simulink model "PIDcontinuo"  (R2021a)
settings: Solver=VariableStepAuto  StartTime=0.0  StopTime=10*ts  RelTol=1e-3
values from neighbouring files (symbols this model uses):
  g = 9.81    [Parcial2PIDContinuo.m]
  L = 0.25    [Parcial2PIDContinuo.m]
  m = 0.03    [Parcial2PIDContinuo.m]
  M = 0.510    (= 0.51)    [Parcial2PIDContinuo.m]
  ts = 5    [Parcial2PIDContinuo.m]
libraries: pid_lib x2, spsStairGeneratorLib x1
settings Model: Creator=manue  LastModifiedBy=manue

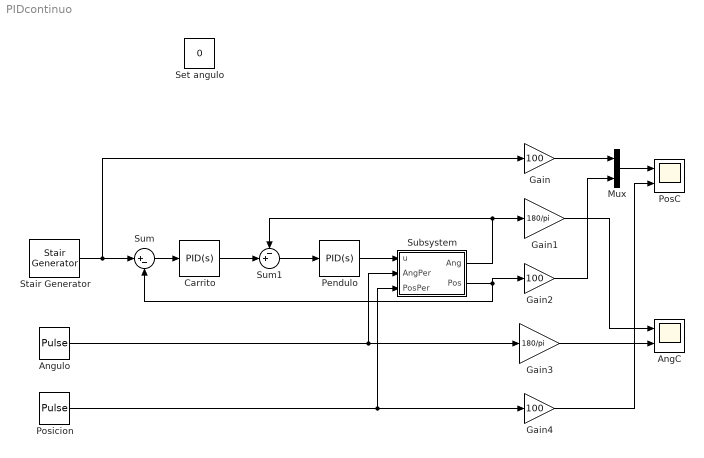
== system PIDcontinuo ==
  AngC : Scope  NumInputPorts=2
  Angulo : DiscretePulseGenerator  PulseType=Time based  Amplitude=10*pi/180  Period=60  PulseWidth=0.1  PhaseDelay=40
  Carrito : pid_lib/PID Controller  Controller=PID  Form=Ideal  TimeDomain=Continuous-time  UseExternalTs=off  SampleTime=-1  IntegratorMethod=Forward Euler  FilterMethod=Forward Euler  ControllerParametersSource=internal  P=0.0857737044561583  I=0.0832220773397635  D=1.96746042698113  UseFilter=on  N=7.47498988089675  TunerSelectOption=Transfer Function Based (PID Tuner App)  InitialConditionSource=internal  InitialConditionForIntegrator=0  InitialConditionForFilter=0  DifferentiatorICPrevScaledInput=0  ExternalReset=none  TrackingMode=off  Kt=1  LimitOutput=off  SatLimitsSource=internal  UpperSaturationLimit=inf  LowerSaturationLimit=-inf  LinearizeAsGain=on  AntiWindupMode=none  Kb=1  POutMin=[]  POutMax=[]  IOutMin=[]  IOutMax=[]  DOutMin=[]  DOutMax=[]  NOutMin=[]  NOutMax=[]  SumOutMin=[]  SumOutMax=[]  SaturationOutMin=[]  SaturationOutMax=[]  PParamMin=[]  PParamMax=[]  IParamMin=[]  IParamMax=[]  DParamMin=[]  DParamMax=[]  NParamMin=[]  NParamMax=[]  KbParamMin=[]  KbParamMax=[]  KtParamMin=[]  KtParamMax=[]  KbOutMin=[]  KbOutMax=[]  KtOutMin=[]  KtOutMax=[]  IntegratorOutMin=[]  IntegratorOutMax=[]  FilterOutMin=[]  FilterOutMax=[]  SumI1OutMin=[]  SumI1OutMax=[]  SumI2OutMin=[]  SumI2OutMax=[]  SumI3OutMin=[]  SumI3OutMax=[]  SumI4OutMin=[]  SumI4OutMax=[]  SumDOutMin=[]  SumDOutMax=[]  DifferentiatorOutMin=[]  DifferentiatorOutMax=[]  FilterDiffOutCoefMin=[]  FilterDiffOutCoefMax=[]  ReciprocalOutMin=[]  ReciprocalOutMax=[]  SumDenOutMin=[]  SumDenOutMax=[]  SumNumOutMin=[]  SumNumOutMax=[]  DivideOutMin=[]  DivideOutMax=[]  UdiffTsProdOutMin=[]  UdiffTsProdOutMax=[]  NTsProdOutMin=[]  NTsProdOutMax=[]  UintegralTsProdOutMin=[]  UintegralTsProdOutMax=[]  UngainTsProdOutMin=[]  UngainTsProdOutMax=[]  IntegratorContinuousStateAttributes=''  IntegratorStateMustResolveToSignalObject=off  IntegratorRTWStateStorageClass=Auto  FilterContinuousStateAttributes=''  FilterStateMustResolveToSignalObject=off  FilterRTWStateStorageClass=Auto  ParallelPVariant=Passthrough  IdealPVariant=InternalParameters  IVariant=InternalParameters  DVariant=InternalParameters  IntegratorVariant=Continuous  SatVariant=Disabled  AWVariant=Passthrough  PCopyVariant=Disabled  TRVariant=Disabled  FdbkBlocksVariant=Forward  IdealPFdbkVariant=Disabled  SatFdbkVariant=Disabled  DerivativeFilterVariant=ContFilter  NVariant=InternalParameters  NCopyVariant=Disabled  FilterICVariant=InternalICsFilter  IntegratorICVariant=InternalICs  ExternalResetVariant=Disabled  TRSumVariant=Passthrough  SumFdbkVariant=Disabled  SumVariant=Sum_PID  TsampFilterVariant=InternalTs  TsampNgainVariant=Passthrough  TsampIntegralVariant=Passthrough  ExternalSaturationOutDataTypeStr=Inherit: Same as second input
  Gain : Gain  Gain=100
  Gain1 : Gain  Gain=180/pi
  Gain2 : Gain  Gain=100
  Gain3 : Gain  Gain=180/pi
  Gain4 : Gain  Gain=100
  Mux : Mux  Inputs=2
  Pendulo : pid_lib/PID Controller  Controller=PID  Form=Ideal  TimeDomain=Continuous-time  UseExternalTs=off  SampleTime=-1  IntegratorMethod=Forward Euler  FilterMethod=Forward Euler  ControllerParametersSource=internal  P=-54.8683679286121  I=2.04775747078051  D=0.0904146272305055  UseFilter=on  N=83.9576991418546  TunerSelectOption=Transfer Function Based (PID Tuner App)  InitialConditionSource=internal  InitialConditionForIntegrator=0  InitialConditionForFilter=0  DifferentiatorICPrevScaledInput=0  ExternalReset=none  TrackingMode=off  Kt=1  LimitOutput=off  SatLimitsSource=internal  UpperSaturationLimit=inf  LowerSaturationLimit=-inf  LinearizeAsGain=on  AntiWindupMode=none  Kb=1  POutMin=[]  POutMax=[]  IOutMin=[]  IOutMax=[]  DOutMin=[]  DOutMax=[]  NOutMin=[]  NOutMax=[]  SumOutMin=[]  SumOutMax=[]  SaturationOutMin=[]  SaturationOutMax=[]  PParamMin=[]  PParamMax=[]  IParamMin=[]  IParamMax=[]  DParamMin=[]  DParamMax=[]  NParamMin=[]  NParamMax=[]  KbParamMin=[]  KbParamMax=[]  KtParamMin=[]  KtParamMax=[]  KbOutMin=[]  KbOutMax=[]  KtOutMin=[]  KtOutMax=[]  IntegratorOutMin=[]  IntegratorOutMax=[]  FilterOutMin=[]  FilterOutMax=[]  SumI1OutMin=[]  SumI1OutMax=[]  SumI2OutMin=[]  SumI2OutMax=[]  SumI3OutMin=[]  SumI3OutMax=[]  SumI4OutMin=[]  SumI4OutMax=[]  SumDOutMin=[]  SumDOutMax=[]  DifferentiatorOutMin=[]  DifferentiatorOutMax=[]  FilterDiffOutCoefMin=[]  FilterDiffOutCoefMax=[]  ReciprocalOutMin=[]  ReciprocalOutMax=[]  SumDenOutMin=[]  SumDenOutMax=[]  SumNumOutMin=[]  SumNumOutMax=[]  DivideOutMin=[]  DivideOutMax=[]  UdiffTsProdOutMin=[]  UdiffTsProdOutMax=[]  NTsProdOutMin=[]  NTsProdOutMax=[]  UintegralTsProdOutMin=[]  UintegralTsProdOutMax=[]  UngainTsProdOutMin=[]  UngainTsProdOutMax=[]  IntegratorContinuousStateAttributes=''  IntegratorStateMustResolveToSignalObject=off  IntegratorRTWStateStorageClass=Auto  FilterContinuousStateAttributes=''  FilterStateMustResolveToSignalObject=off  FilterRTWStateStorageClass=Auto  ParallelPVariant=Passthrough  IdealPVariant=InternalParameters  IVariant=InternalParameters  DVariant=InternalParameters  IntegratorVariant=Continuous  SatVariant=Disabled  AWVariant=Passthrough  PCopyVariant=Disabled  TRVariant=Disabled  FdbkBlocksVariant=Forward  IdealPFdbkVariant=Disabled  SatFdbkVariant=Disabled  DerivativeFilterVariant=ContFilter  NVariant=InternalParameters  NCopyVariant=Disabled  FilterICVariant=InternalICsFilter  IntegratorICVariant=InternalICs  ExternalResetVariant=Disabled  TRSumVariant=Passthrough  SumFdbkVariant=Disabled  SumVariant=Sum_PID  TsampFilterVariant=InternalTs  TsampNgainVariant=Passthrough  TsampIntegralVariant=Passthrough  ExternalSaturationOutDataTypeStr=Inherit: Same as second input
  PosC : Scope  NumInputPorts=2
  Posicion : DiscretePulseGenerator  PulseType=Time based  Amplitude=5/100  Period=60  PhaseDelay=20
  Set angulo : Constant  Value=0
  Stair Generator : spsStairGeneratorLib/Stair Generator  t=[0, ts,2*ts,3*ts,4*ts,5*ts,6*ts,7*ts,8*ts,9*ts,10*ts]  e=[25,35,35,40,40,35,35,10,10,30,30]/100  Ts=0
  Subsystem : Subsystem
  Sum : Sum  Inputs=|+-
  Sum1 : Sum  Inputs=-+|
  wires:
  Sum/1 -> Carrito/1
  Gain/1 -> Mux/1
  Gain2/1 -> Mux/2
  Mux/1 -> PosC/1
  Gain4/1 -> PosC/2
  Gain3/1 -> AngC/2
  Gain1/1 -> AngC/1
  Stair Generator/1 -> Gain/1, Sum/1
  Sum1/1 -> Pendulo/1
  Posicion/1 -> Subsystem/3(PosPer), Gain4/1
  Subsystem/1(Ang) -> Sum1/1, Gain1/1
  Subsystem/2(Pos) -> Gain2/1, Sum/2
  Angulo/1 -> Subsystem/2(AngPer), Gain3/1
  Pendulo/1 -> Subsystem/1(u)
  Carrito/1 -> Sum1/2

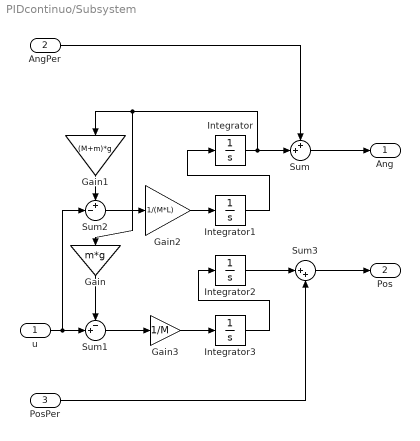
== system PIDcontinuo/Subsystem ==
  u : Inport
  AngPer : Inport  Port=2
  PosPer : Inport  Port=3
  Gain : Gain  Gain=m*g
  Gain1 : Gain  Gain=(M+m)*g
  Gain2 : Gain  Gain=1/(M*L)
  Gain3 : Gain  Gain=1/M
  Integrator : Integrator  InitialCondition=10*pi/180
  Integrator1 : Integrator
  Integrator2 : Integrator
  Integrator3 : Integrator
  Sum : Sum  Inputs=++|
  Sum1 : Sum  Inputs=-+|
  Sum2 : Sum  Inputs=+-|
  Sum3 : Sum  Inputs=|++
  Ang : Outport
  Pos : Outport  Port=2
  wires:
  AngPer/1 -> Sum/1
  Integrator/1 -> Gain1/1, Gain/1, Sum/2
  Gain/1 -> Sum1/1
  Gain1/1 -> Sum2/1
  u/1 -> Sum2/2, Sum1/2
  Sum2/1 -> Gain2/1
  Gain2/1 -> Integrator1/1
  Integrator1/1 -> Integrator/1
  Sum1/1 -> Gain3/1
  Gain3/1 -> Integrator3/1
  Integrator3/1 -> Integrator2/1
  Integrator2/1 -> Sum3/1
  PosPer/1 -> Sum3/2
  Sum3/1 -> Pos/1
  Sum/1 -> Ang/1
